simulink model "Lab1_NomPlantModel_2018a"  (R2018a)
settings: Solver=VariableStepAuto  StartTime=0.0  StopTime=100  RelTol=1e-3
libraries: cstblocks x1
settings Model: Creator=emma  LastModifiedBy=emma
settings DataIOCC: ReturnWorkspaceOutputs=on
settings SFSimCC: SimUseLocalCustomCode=on
settings RTWCC: RTWUseLocalCustomCode=on

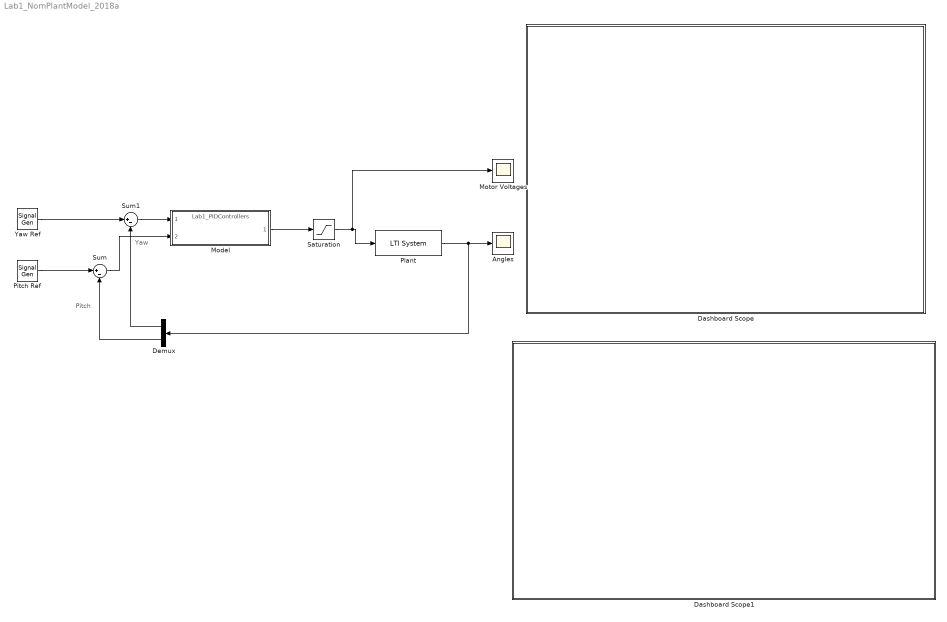
== system Lab1_NomPlantModel_2018a ==
  note: Yaw
  note: Pitch
  Angles : Scope
  Dashboard Scope : Subsystem  DialogController=hmiCreateDDGDialog  IsWebBlock=on  mask(MWDashboardBlock){webBlockId=999f5c87-4258-4756-b441-ab429ee74347, webBlockType=sdiscope, ShowInLibBrowser=on, ShowInitialText=on, HMISrcModelName=Lab1_NomPlantModel_2018a}
      mask prompts: webBlockId "WebBlock Id"; webBlockType "WebBlock Type"; HMISrcModelName "Source Model"
      mask help: Traces signals on the dashboard scope during simulation.
      mask Help: helpview([docroot '/mapfiles/simulink.map'], 'hmi_scope')
      mask Display:
      | if strcmp(get_param(bdroot(gcb),'BlockDiagramType'),'library')
      |  image([(matlabroot) '/toolbox/simulink/hmi/icons/SDIScope.png'])
      | end
  Dashboard Scope1 : Subsystem  DialogController=hmiCreateDDGDialog  IsWebBlock=on  mask(MWDashboardBlock){webBlockId=d35f1527-02ee-476e-a039-b9c737d0bbbb, webBlockType=sdiscope, ShowInLibBrowser=on, ShowInitialText=on, HMISrcModelName=Lab1_NomPlantModel_2018a}
      mask prompts: webBlockId "WebBlock Id"; webBlockType "WebBlock Type"; HMISrcModelName "Source Model"
      mask help: Traces signals on the dashboard scope during simulation.
      mask Help: helpview([docroot '/mapfiles/simulink.map'], 'hmi_scope')
      mask Display:
      | if strcmp(get_param(bdroot(gcb),'BlockDiagramType'),'library')
      |  image([(matlabroot) '/toolbox/simulink/hmi/icons/SDIScope.png'])
      | end
  Demux : Demux  Outputs=2
  Model : ModelReference  ModelNameDialog=Lab1_PIDControllers.slx  SimulationMode=Normal  ModelReferenceVersion=1.2
  Motor Voltages : Scope
  Pitch Ref : SignalGenerator  WaveForm=square  Amplitude=pi/6  Frequency=0.4  Units=rad/sec
  Plant : cstblocks/LTI System  sys=Gnom  IC=[]
  Saturation : Saturate  UpperLimit=+25  LowerLimit=-25
  Sum : Sum  Inputs=|+-
  Sum1 : Sum  Inputs=|+-
  Yaw Ref : SignalGenerator  WaveForm=square  Amplitude=pi/4  Frequency=0.5  Units=rad/sec
  wires:
  Yaw Ref/1 -> Sum1/1
  Plant/1 -> Demux/1, Angles/1
  Pitch Ref/1 -> Sum/1
  Demux/1 -> Sum1/2
  Demux/2 -> Sum/2
  Sum1/1 -> Model/1
  Sum/1 -> Model/2
  Model/1 -> Saturation/1
  Saturation/1 -> Motor Voltages/1, Plant/1

== system Lab1_NomPlantModel_2018a/Dashboard Scope ==

== system Lab1_NomPlantModel_2018a/Dashboard Scope1 ==
